simulink model "npc_controller"  (R2022a)
settings: Solver=FixedStepDiscrete  StartTime=0.0  StopTime=20  RelTol=1e-3  EnableMultiTasking=on
values from neighbouring files (symbols this model uses):
  Tsw = 1.5E-5    [param.sldd]
undefined symbols (not defined in the file or in its folder): CAN_O_INT, CANA_BASE, Down, GPTRIP1SEL, GPTRIP2SEL, GPTRIP3SEL, TZ1, TZ2, TZ3, Up
libraries: simulink x153, hdlsllib x90, c2802xlib x34, c2837xDlib x18, c280xlib x12, canmsglib x9, c2838xlib x8, idelinklib_common x3, c2806xlib x2, slpidlib x2, c28004xlib x2, c281xlib x2
(part 39 of 45)

== system npc_controller/IDLE_AND_TIMER/codegen/IDLE/idle_task/report_adc/Subsystem8 ==
  adc : Inport
  zero_offset : Inport  Port=2
  gain : Inport  Port=3
  Product6 : Product  OutDataTypeStr=single
  Saturation : Saturate  UpperLimit=inf  LowerLimit=0
  Subtract : Sum  Inputs=+-  AccumDataTypeStr=single  OutDataTypeStr=single
  actual : Outport
  wires:
  Saturation/1 -> Product6/1
  Subtract/1 -> Saturation/1
  zero_offset/1 -> Subtract/2
  adc/1 -> Subtract/1
  gain/1 -> Product6/2
  Product6/1 -> actual/1

== system npc_controller/IDLE_AND_TIMER/codegen/IDLE/idle_task/report_adc/Subsystem9 ==
  adc : Inport
  gain : Inport  Port=2
  Product6 : Product  OutDataTypeStr=single
  actual : Outport
  wires:
  adc/1 -> Product6/1
  gain/1 -> Product6/2
  Product6/1 -> actual/1

== system npc_controller/IDLE_AND_TIMER/codegen/IDLE/idle_task/report_adc1/Subsystem1 ==
  adc : Inport
  zero_offset : Inport  Port=2
  gain : Inport  Port=3
  Product6 : Product  OutDataTypeStr=single
  Saturation : Saturate  UpperLimit=inf  LowerLimit=0
  Subtract : Sum  Inputs=+-  AccumDataTypeStr=single  OutDataTypeStr=single
  actual : Outport
  wires:
  Product6/1 -> actual/1
  gain/1 -> Product6/2
  adc/1 -> Subtract/1
  zero_offset/1 -> Subtract/2
  Subtract/1 -> Saturation/1
  Saturation/1 -> Product6/1

== system npc_controller/IDLE_AND_TIMER/codegen/IDLE/idle_task/report_adc1/Subsystem10 ==
  adc : Inport
  gain : Inport  Port=2
  Product6 : Product  OutDataTypeStr=single
  actual : Outport
  wires:
  adc/1 -> Product6/1
  gain/1 -> Product6/2
  Product6/1 -> actual/1

== system npc_controller/IDLE_AND_TIMER/codegen/IDLE/idle_task/report_adc1/Subsystem11 ==
  adc : Inport
  zero_offset : Inport  Port=2
  gain : Inport  Port=3
  Product6 : Product  OutDataTypeStr=single
  Saturation : Saturate  UpperLimit=inf  LowerLimit=0
  Subtract : Sum  Inputs=+-  AccumDataTypeStr=single  OutDataTypeStr=single
  actual : Outport
  wires:
  Saturation/1 -> Product6/1
  Subtract/1 -> Saturation/1
  zero_offset/1 -> Subtract/2
  adc/1 -> Subtract/1
  gain/1 -> Product6/2
  Product6/1 -> actual/1

== system npc_controller/IDLE_AND_TIMER/codegen/IDLE/idle_task/report_adc1/Subsystem2 ==
  adc : Inport
  zero_offset : Inport  Port=2
  gain : Inport  Port=3
  Product6 : Product  OutDataTypeStr=single
  Saturation : Saturate  UpperLimit=inf  LowerLimit=0
  Subtract : Sum  Inputs=+-  AccumDataTypeStr=single  OutDataTypeStr=single
  actual : Outport
  wires:
  Saturation/1 -> Product6/1
  Subtract/1 -> Saturation/1
  zero_offset/1 -> Subtract/2
  adc/1 -> Subtract/1
  gain/1 -> Product6/2
  Product6/1 -> actual/1

== system npc_controller/IDLE_AND_TIMER/codegen/IDLE/idle_task/report_adc1/Subsystem3 ==
  adc : Inport
  zero_offset : Inport  Port=2
  gain : Inport  Port=3
  Product6 : Product  OutDataTypeStr=single
  Saturation : Saturate  UpperLimit=inf  LowerLimit=0
  Subtract : Sum  Inputs=+-  AccumDataTypeStr=single  OutDataTypeStr=single
  actual : Outport
  wires:
  Product6/1 -> actual/1
  gain/1 -> Product6/2
  adc/1 -> Subtract/1
  zero_offset/1 -> Subtract/2
  Subtract/1 -> Saturation/1
  Saturation/1 -> Product6/1

== system npc_controller/IDLE_AND_TIMER/codegen/IDLE/idle_task/report_adc1/Subsystem4 ==
  adc : Inport
  zero_offset : Inport  Port=2
  gain : Inport  Port=3
  Product6 : Product  OutDataTypeStr=single
  Saturation : Saturate  UpperLimit=inf  LowerLimit=0
  Subtract : Sum  Inputs=+-  AccumDataTypeStr=single  OutDataTypeStr=single
  actual : Outport
  wires:
  Saturation/1 -> Product6/1
  Subtract/1 -> Saturation/1
  zero_offset/1 -> Subtract/2
  adc/1 -> Subtract/1
  gain/1 -> Product6/2
  Product6/1 -> actual/1

== system npc_controller/IDLE_AND_TIMER/codegen/IDLE/idle_task/report_adc1/Subsystem5 ==
  adc : Inport
  zero_offset : Inport  Port=2
  gain : Inport  Port=3
  Product6 : Product  OutDataTypeStr=single
  Saturation : Saturate  UpperLimit=inf  LowerLimit=0
  Subtract : Sum  Inputs=+-  AccumDataTypeStr=single  OutDataTypeStr=single
  actual : Outport
  wires:
  Product6/1 -> actual/1
  gain/1 -> Product6/2
  adc/1 -> Subtract/1
  zero_offset/1 -> Subtract/2
  Subtract/1 -> Saturation/1
  Saturation/1 -> Product6/1

== system npc_controller/IDLE_AND_TIMER/codegen/IDLE/idle_task/report_adc1/Subsystem6 ==
  adc : Inport
  zero_offset : Inport  Port=2
  gain : Inport  Port=3
  Product6 : Product  OutDataTypeStr=single
  Saturation : Saturate  UpperLimit=inf  LowerLimit=0
  Subtract : Sum  Inputs=+-  AccumDataTypeStr=single  OutDataTypeStr=single
  actual : Outport
  wires:
  Saturation/1 -> Product6/1
  Subtract/1 -> Saturation/1
  zero_offset/1 -> Subtract/2
  adc/1 -> Subtract/1
  gain/1 -> Product6/2
  Product6/1 -> actual/1

== system npc_controller/IDLE_AND_TIMER/codegen/IDLE/idle_task/report_adc1/Subsystem7 ==
  adc : Inport
  zero_offset : Inport  Port=2
  gain : Inport  Port=3
  Product6 : Product  OutDataTypeStr=single
  Saturation : Saturate  UpperLimit=inf  LowerLimit=0
  Subtract : Sum  Inputs=+-  AccumDataTypeStr=single  OutDataTypeStr=single
  actual : Outport
  wires:
  Saturation/1 -> Product6/1
  Subtract/1 -> Saturation/1
  zero_offset/1 -> Subtract/2
  adc/1 -> Subtract/1
  gain/1 -> Product6/2
  Product6/1 -> actual/1

== system npc_controller/IDLE_AND_TIMER/codegen/IDLE/idle_task/report_adc1/Subsystem8 ==
  adc : Inport
  zero_offset : Inport  Port=2
  gain : Inport  Port=3
  Product6 : Product  OutDataTypeStr=single
  Saturation : Saturate  UpperLimit=inf  LowerLimit=0
  Subtract : Sum  Inputs=+-  AccumDataTypeStr=single  OutDataTypeStr=single
  actual : Outport
  wires:
  Product6/1 -> actual/1
  gain/1 -> Product6/2
  adc/1 -> Subtract/1
  zero_offset/1 -> Subtract/2
  Subtract/1 -> Saturation/1
  Saturation/1 -> Product6/1

== system npc_controller/IDLE_AND_TIMER/codegen/IDLE/idle_task/report_adc1/Subsystem9 ==
  adc : Inport
  gain : Inport  Port=2
  Product6 : Product  OutDataTypeStr=single
  actual : Outport
  wires:
  Product6/1 -> actual/1
  gain/1 -> Product6/2
  adc/1 -> Product6/1

== system npc_controller/IDLE_AND_TIMER/codegen/IDLE/idle_task/set_tmp_mux/incr_cnt_tmp_mux ==
  function : TriggerPort  TriggerType=function-call  VariantControl=Variant
  Data Store Read : DataStoreRead  DataStoreName=cnt_tmp_mux  IndexOptions=Index vector (dialog)  Indices=1  OutputSizes=1
  If : If  IfExpression=u1 < 4
  cnt_idle : Subsystem  TreatAsAtomicUnit=on
  cnt_idle_sat : Subsystem  TreatAsAtomicUnit=on
  wires:
  Data Store Read/1 -> If/1
  If/1 -> cnt_idle/Action
  If/2 -> cnt_idle_sat/Action

== system npc_controller/IDLE_AND_TIMER/codegen/IDLE/idle_task/set_tmp_mux/parse_cnt_tmp_mux ==
  function : TriggerPort  TriggerType=function-call  VariantControl=Variant
  Data Store Read : DataStoreRead  DataStoreName=cnt_tmp_mux  IndexOptions=Index vector (dialog)  Indices=1  OutputSizes=1
  Switch Case : SwitchCase  CaseConditions={0, 1, 2, 3}
  cnt_tmp_mux_0 : Subsystem  TreatAsAtomicUnit=on
  cnt_tmp_mux_1 : Subsystem  TreatAsAtomicUnit=on
  cnt_tmp_mux_2 : Subsystem  TreatAsAtomicUnit=on
  cnt_tmp_mux_3 : Subsystem  TreatAsAtomicUnit=on
  wires:
  Data Store Read/1 -> Switch Case/1
  Switch Case/1 -> cnt_tmp_mux_0/Action
  Switch Case/2 -> cnt_tmp_mux_1/Action
  Switch Case/3 -> cnt_tmp_mux_2/Action
  Switch Case/4 -> cnt_tmp_mux_3/Action

== system npc_controller/IDLE_AND_TIMER/codegen/IDLE/idle_task/set_tmp_mux/set_tmp_mux ==
  Trigger : TriggerPort  TriggerType=function-call  VariantControl=(inherit)  PortDimensions=1
  Data Store Read : DataStoreRead  DataStoreName=tmp_mux_s0  IndexOptions=Index vector (dialog)  Indices=1  OutputSizes=1
  Data Store Read1 : DataStoreRead  DataStoreName=tmp_mux_s1  IndexOptions=Index vector (dialog)  Indices=1  OutputSizes=1
  Data Store Read2 : DataStoreRead  DataStoreName=tmp_mux_s2  IndexOptions=Index vector (dialog)  Indices=1  OutputSizes=1
  GPIO63 : c2837xDlib/Digital Output  GPIO_Number=GPIO56~GPIO63  GPIO_Bit0=off  GPIO_BIT0_Toggle=off  GPIO_Bit1=off  GPIO_BIT1_Toggle=off  GPIO_Bit2=off  GPIO_BIT2_Toggle=off  GPIO_Bit3=off  GPIO_BIT3_Toggle=off  GPIO_Bit4=off  GPIO_BIT4_Toggle=off  GPIO_Bit5=off  GPIO_BIT5_Toggle=off  GPIO_Bit6=off  GPIO_BIT6_Toggle=off  GPIO_Bit7=on  GPIO_BIT7_Toggle=off
      settings: SourceProductBaseCode=TIC2000
  GPIO64 : c2837xDlib/Digital Output  GPIO_Number=GPIO64~GPIO71  GPIO_Bit0=on  GPIO_BIT0_Toggle=off  GPIO_Bit1=off  GPIO_BIT1_Toggle=off  GPIO_Bit2=off  GPIO_BIT2_Toggle=off  GPIO_Bit3=off  GPIO_BIT3_Toggle=off  GPIO_Bit4=off  GPIO_BIT4_Toggle=off  GPIO_Bit5=off  GPIO_BIT5_Toggle=off  GPIO_Bit6=off  GPIO_BIT6_Toggle=off  GPIO_Bit7=off  GPIO_BIT7_Toggle=off
      settings: SourceProductBaseCode=TIC2000
  GPIO65 : c2837xDlib/Digital Output  GPIO_Number=GPIO64~GPIO71  GPIO_Bit0=off  GPIO_BIT0_Toggle=off  GPIO_Bit1=on  GPIO_BIT1_Toggle=off  GPIO_Bit2=off  GPIO_BIT2_Toggle=off  GPIO_Bit3=off  GPIO_BIT3_Toggle=off  GPIO_Bit4=off  GPIO_BIT4_Toggle=off  GPIO_Bit5=off  GPIO_BIT5_Toggle=off  GPIO_Bit6=off  GPIO_BIT6_Toggle=off  GPIO_Bit7=off  GPIO_BIT7_Toggle=off
      settings: SourceProductBaseCode=TIC2000
  wires:
  Data Store Read1/1 -> GPIO64/1
  Data Store Read/1 -> GPIO63/1
  Data Store Read2/1 -> GPIO65/1

== system npc_controller/IDLE_AND_TIMER/codegen/IDLE/idle_task1/get_adc_tmp_mux/get_tmp_mux_inlet ==
  In1 : Inport
  Action Port : ActionPort  ActionPortLabel=case [ 3 ]:
  Data Store Write13 : DataStoreWrite  DataStoreName=adc_temp_inlet  IndexOptions=Index vector (dialog)  Indices=1  OutputSizes=1
  wires:
  In1/1 -> Data Store Write13/1

== system npc_controller/IDLE_AND_TIMER/codegen/IDLE/idle_task1/get_adc_tmp_mux/get_tmp_mux_npca ==
  In1 : Inport
  Action Port : ActionPort  ActionPortLabel=case [ 0 ]:
  Data Store Write13 : DataStoreWrite  DataStoreName=adc_temp_npca  IndexOptions=Index vector (dialog)  Indices=1  OutputSizes=1
  wires:
  In1/1 -> Data Store Write13/1

== system npc_controller/IDLE_AND_TIMER/codegen/IDLE/idle_task1/get_adc_tmp_mux/get_tmp_mux_npcb ==
  In1 : Inport
  Action Port : ActionPort  ActionPortLabel=case [ 1 ]:
  Data Store Write13 : DataStoreWrite  DataStoreName=adc_temp_npcb  IndexOptions=Index vector (dialog)  Indices=1  OutputSizes=1
  wires:
  In1/1 -> Data Store Write13/1

== system npc_controller/IDLE_AND_TIMER/codegen/IDLE/idle_task1/get_adc_tmp_mux/get_tmp_mux_npcc ==
  In1 : Inport
  Action Port : ActionPort  ActionPortLabel=case [ 2 ]:
  Data Store Write13 : DataStoreWrite  DataStoreName=adc_temp_npcc  IndexOptions=Index vector (dialog)  Indices=1  OutputSizes=1
  wires:
  In1/1 -> Data Store Write13/1

== system npc_controller/IDLE_AND_TIMER/codegen/IDLE/idle_task1/hkeep/tfv ==
  function : TriggerPort  TriggerType=function-call  VariantControl=Variant
  hkeep1 : Stateflow chart  TreatAsAtomicUnit=on

== system npc_controller/IDLE_AND_TIMER/codegen/IDLE/idle_task1/hkeep/tz ==
  note: reading the tz flag through epwm2 registers and writing to tz_ocp and tz_ovp variables. tz_ocp & tz_ovp are used in state machine
  note: npc_controller_DWork .tz_ocp = EPwm2Regs.TZOSTFLG.bit.OST1;
      | npc_controller_DWork .tz_ovp = EPwm2Regs.TZOSTFLG.bit.OST2;
  function : TriggerPort  TriggerType=function-call  VariantControl=Variant
  System Outputs2 : Subsystem  mask(System Outputs){ShowInLibBrowser=0}
      mask prompts: ShowInLibBrowser "Simulink:masks:CustCodeMaskParam1_MP"
      settings: CopyFcn=cccopyfcn(gcb)  OpenFcn=ccopenfcn('System Outputs Function')
      mask Help: eval('feval(''rtwprivate'',''rtwhelpview'',''rtw_sys_outputs_block'')');
      mask Display: disp('System\nOutputs');

== system npc_controller/IDLE_AND_TIMER/codegen/IDLE/idle_task1/report_adc/Subsystem1 ==
  adc : Inport
  zero_offset : Inport  Port=2
  gain : Inport  Port=3
  Product6 : Product  OutDataTypeStr=single
  Saturation : Saturate  UpperLimit=inf  LowerLimit=0
  Subtract : Sum  Inputs=+-  AccumDataTypeStr=single  OutDataTypeStr=single
  actual : Outport
  wires:
  Saturation/1 -> Product6/1
  Subtract/1 -> Saturation/1
  zero_offset/1 -> Subtract/2
  adc/1 -> Subtract/1
  gain/1 -> Product6/2
  Product6/1 -> actual/1

== system npc_controller/IDLE_AND_TIMER/codegen/IDLE/idle_task1/report_adc/Subsystem10 ==
  adc : Inport
  gain : Inport  Port=2
  Product6 : Product  OutDataTypeStr=single
  actual : Outport
  wires:
  Product6/1 -> actual/1
  gain/1 -> Product6/2
  adc/1 -> Product6/1

== system npc_controller/IDLE_AND_TIMER/codegen/IDLE/idle_task1/report_adc/Subsystem11 ==
  adc : Inport
  zero_offset : Inport  Port=2
  gain : Inport  Port=3
  Product6 : Product  OutDataTypeStr=single
  Saturation : Saturate  UpperLimit=inf  LowerLimit=0
  Subtract : Sum  Inputs=+-  AccumDataTypeStr=single  OutDataTypeStr=single
  actual : Outport
  wires:
  Product6/1 -> actual/1
  gain/1 -> Product6/2
  adc/1 -> Subtract/1
  zero_offset/1 -> Subtract/2
  Subtract/1 -> Saturation/1
  Saturation/1 -> Product6/1

== system npc_controller/IDLE_AND_TIMER/codegen/IDLE/idle_task1/report_adc/Subsystem2 ==
  adc : Inport
  zero_offset : Inport  Port=2
  gain : Inport  Port=3
  Product6 : Product  OutDataTypeStr=single
  Saturation : Saturate  UpperLimit=inf  LowerLimit=0
  Subtract : Sum  Inputs=+-  AccumDataTypeStr=single  OutDataTypeStr=single
  actual : Outport
  wires:
  Product6/1 -> actual/1
  gain/1 -> Product6/2
  adc/1 -> Subtract/1
  zero_offset/1 -> Subtract/2
  Subtract/1 -> Saturation/1
  Saturation/1 -> Product6/1

== system npc_controller/IDLE_AND_TIMER/codegen/IDLE/idle_task1/report_adc/Subsystem3 ==
  adc : Inport
  zero_offset : Inport  Port=2
  gain : Inport  Port=3
  Product6 : Product  OutDataTypeStr=single
  Saturation : Saturate  UpperLimit=inf  LowerLimit=0
  Subtract : Sum  Inputs=+-  AccumDataTypeStr=single  OutDataTypeStr=single
  actual : Outport
  wires:
  Saturation/1 -> Product6/1
  Subtract/1 -> Saturation/1
  zero_offset/1 -> Subtract/2
  adc/1 -> Subtract/1
  gain/1 -> Product6/2
  Product6/1 -> actual/1

== system npc_controller/IDLE_AND_TIMER/codegen/IDLE/idle_task1/report_adc/Subsystem4 ==
  adc : Inport
  zero_offset : Inport  Port=2
  gain : Inport  Port=3
  Product6 : Product  OutDataTypeStr=single
  Saturation : Saturate  UpperLimit=inf  LowerLimit=0
  Subtract : Sum  Inputs=+-  AccumDataTypeStr=single  OutDataTypeStr=single
  actual : Outport
  wires:
  Product6/1 -> actual/1
  gain/1 -> Product6/2
  adc/1 -> Subtract/1
  zero_offset/1 -> Subtract/2
  Subtract/1 -> Saturation/1
  Saturation/1 -> Product6/1

== system npc_controller/IDLE_AND_TIMER/codegen/IDLE/idle_task1/report_adc/Subsystem5 ==
  adc : Inport
  zero_offset : Inport  Port=2
  gain : Inport  Port=3
  Product6 : Product  OutDataTypeStr=single
  Saturation : Saturate  UpperLimit=inf  LowerLimit=0
  Subtract : Sum  Inputs=+-  AccumDataTypeStr=single  OutDataTypeStr=single
  actual : Outport
  wires:
  Saturation/1 -> Product6/1
  Subtract/1 -> Saturation/1
  zero_offset/1 -> Subtract/2
  adc/1 -> Subtract/1
  gain/1 -> Product6/2
  Product6/1 -> actual/1

== system npc_controller/IDLE_AND_TIMER/codegen/IDLE/idle_task1/report_adc/Subsystem6 ==
  adc : Inport
  zero_offset : Inport  Port=2
  gain : Inport  Port=3
  Product6 : Product  OutDataTypeStr=single
  Saturation : Saturate  UpperLimit=inf  LowerLimit=0
  Subtract : Sum  Inputs=+-  AccumDataTypeStr=single  OutDataTypeStr=single
  actual : Outport
  wires:
  Product6/1 -> actual/1
  gain/1 -> Product6/2
  adc/1 -> Subtract/1
  zero_offset/1 -> Subtract/2
  Subtract/1 -> Saturation/1
  Saturation/1 -> Product6/1

== system npc_controller/IDLE_AND_TIMER/codegen/IDLE/idle_task1/report_adc/Subsystem7 ==
  adc : Inport
  zero_offset : Inport  Port=2
  gain : Inport  Port=3
  Product6 : Product  OutDataTypeStr=single
  Saturation : Saturate  UpperLimit=inf  LowerLimit=0
  Subtract : Sum  Inputs=+-  AccumDataTypeStr=single  OutDataTypeStr=single
  actual : Outport
  wires:
  Product6/1 -> actual/1
  gain/1 -> Product6/2
  adc/1 -> Subtract/1
  zero_offset/1 -> Subtract/2
  Subtract/1 -> Saturation/1
  Saturation/1 -> Product6/1

== system npc_controller/IDLE_AND_TIMER/codegen/IDLE/idle_task1/report_adc/Subsystem8 ==
  adc : Inport
  zero_offset : Inport  Port=2
  gain : Inport  Port=3
  Product6 : Product  OutDataTypeStr=single
  Saturation : Saturate  UpperLimit=inf  LowerLimit=0
  Subtract : Sum  Inputs=+-  AccumDataTypeStr=single  OutDataTypeStr=single
  actual : Outport
  wires:
  Saturation/1 -> Product6/1
  Subtract/1 -> Saturation/1
  zero_offset/1 -> Subtract/2
  adc/1 -> Subtract/1
  gain/1 -> Product6/2
  Product6/1 -> actual/1

== system npc_controller/IDLE_AND_TIMER/codegen/IDLE/idle_task1/report_adc/Subsystem9 ==
  adc : Inport
  gain : Inport  Port=2
  Product6 : Product  OutDataTypeStr=single
  actual : Outport
  wires:
  adc/1 -> Product6/1
  gain/1 -> Product6/2
  Product6/1 -> actual/1

== system npc_controller/IDLE_AND_TIMER/codegen/IDLE/idle_task1/report_adc1/Subsystem1 ==
  adc : Inport
  zero_offset : Inport  Port=2
  gain : Inport  Port=3
  Product6 : Product  OutDataTypeStr=single
  Saturation : Saturate  UpperLimit=inf  LowerLimit=0
  Subtract : Sum  Inputs=+-  AccumDataTypeStr=single  OutDataTypeStr=single
  actual : Outport
  wires:
  Product6/1 -> actual/1
  gain/1 -> Product6/2
  adc/1 -> Subtract/1
  zero_offset/1 -> Subtract/2
  Subtract/1 -> Saturation/1
  Saturation/1 -> Product6/1

== system npc_controller/IDLE_AND_TIMER/codegen/IDLE/idle_task1/report_adc1/Subsystem10 ==
  adc : Inport
  gain : Inport  Port=2
  Product6 : Product  OutDataTypeStr=single
  actual : Outport
  wires:
  adc/1 -> Product6/1
  gain/1 -> Product6/2
  Product6/1 -> actual/1

== system npc_controller/IDLE_AND_TIMER/codegen/IDLE/idle_task1/report_adc1/Subsystem11 ==
  adc : Inport
  zero_offset : Inport  Port=2
  gain : Inport  Port=3
  Product6 : Product  OutDataTypeStr=single
  Saturation : Saturate  UpperLimit=inf  LowerLimit=0
  Subtract : Sum  Inputs=+-  AccumDataTypeStr=single  OutDataTypeStr=single
  actual : Outport
  wires:
  Saturation/1 -> Product6/1
  Subtract/1 -> Saturation/1
  zero_offset/1 -> Subtract/2
  adc/1 -> Subtract/1
  gain/1 -> Product6/2
  Product6/1 -> actual/1

== system npc_controller/IDLE_AND_TIMER/codegen/IDLE/idle_task1/report_adc1/Subsystem2 ==
  adc : Inport
  zero_offset : Inport  Port=2
  gain : Inport  Port=3
  Product6 : Product  OutDataTypeStr=single
  Saturation : Saturate  UpperLimit=inf  LowerLimit=0
  Subtract : Sum  Inputs=+-  AccumDataTypeStr=single  OutDataTypeStr=single
  actual : Outport
  wires:
  Saturation/1 -> Product6/1
  Subtract/1 -> Saturation/1
  zero_offset/1 -> Subtract/2
  adc/1 -> Subtract/1
  gain/1 -> Product6/2
  Product6/1 -> actual/1

== system npc_controller/IDLE_AND_TIMER/codegen/IDLE/idle_task1/report_adc1/Subsystem3 ==
  adc : Inport
  zero_offset : Inport  Port=2
  gain : Inport  Port=3
  Product6 : Product  OutDataTypeStr=single
  Saturation : Saturate  UpperLimit=inf  LowerLimit=0
  Subtract : Sum  Inputs=+-  AccumDataTypeStr=single  OutDataTypeStr=single
  actual : Outport
  wires:
  Product6/1 -> actual/1
  gain/1 -> Product6/2
  adc/1 -> Subtract/1
  zero_offset/1 -> Subtract/2
  Subtract/1 -> Saturation/1
  Saturation/1 -> Product6/1

== system npc_controller/IDLE_AND_TIMER/codegen/IDLE/idle_task1/report_adc1/Subsystem4 ==
  adc : Inport
  zero_offset : Inport  Port=2
  gain : Inport  Port=3
  Product6 : Product  OutDataTypeStr=single
  Saturation : Saturate  UpperLimit=inf  LowerLimit=0
  Subtract : Sum  Inputs=+-  AccumDataTypeStr=single  OutDataTypeStr=single
  actual : Outport
  wires:
  Saturation/1 -> Product6/1
  Subtract/1 -> Saturation/1
  zero_offset/1 -> Subtract/2
  adc/1 -> Subtract/1
  gain/1 -> Product6/2
  Product6/1 -> actual/1

== system npc_controller/IDLE_AND_TIMER/codegen/IDLE/idle_task1/report_adc1/Subsystem5 ==
  adc : Inport
  zero_offset : Inport  Port=2
  gain : Inport  Port=3
  Product6 : Product  OutDataTypeStr=single
  Saturation : Saturate  UpperLimit=inf  LowerLimit=0
  Subtract : Sum  Inputs=+-  AccumDataTypeStr=single  OutDataTypeStr=single
  actual : Outport
  wires:
  Product6/1 -> actual/1
  gain/1 -> Product6/2
  adc/1 -> Subtract/1
  zero_offset/1 -> Subtract/2
  Subtract/1 -> Saturation/1
  Saturation/1 -> Product6/1

== system npc_controller/IDLE_AND_TIMER/codegen/IDLE/idle_task1/report_adc1/Subsystem6 ==
  adc : Inport
  zero_offset : Inport  Port=2
  gain : Inport  Port=3
  Product6 : Product  OutDataTypeStr=single
  Saturation : Saturate  UpperLimit=inf  LowerLimit=0
  Subtract : Sum  Inputs=+-  AccumDataTypeStr=single  OutDataTypeStr=single
  actual : Outport
  wires:
  Saturation/1 -> Product6/1
  Subtract/1 -> Saturation/1
  zero_offset/1 -> Subtract/2
  adc/1 -> Subtract/1
  gain/1 -> Product6/2
  Product6/1 -> actual/1

== system npc_controller/IDLE_AND_TIMER/codegen/IDLE/idle_task1/report_adc1/Subsystem7 ==
  adc : Inport
  zero_offset : Inport  Port=2
  gain : Inport  Port=3
  Product6 : Product  OutDataTypeStr=single
  Saturation : Saturate  UpperLimit=inf  LowerLimit=0
  Subtract : Sum  Inputs=+-  AccumDataTypeStr=single  OutDataTypeStr=single
  actual : Outport
  wires:
  Saturation/1 -> Product6/1
  Subtract/1 -> Saturation/1
  zero_offset/1 -> Subtract/2
  adc/1 -> Subtract/1
  gain/1 -> Product6/2
  Product6/1 -> actual/1

== system npc_controller/IDLE_AND_TIMER/codegen/IDLE/idle_task1/report_adc1/Subsystem8 ==
  adc : Inport
  zero_offset : Inport  Port=2
  gain : Inport  Port=3
  Product6 : Product  OutDataTypeStr=single
  Saturation : Saturate  UpperLimit=inf  LowerLimit=0
  Subtract : Sum  Inputs=+-  AccumDataTypeStr=single  OutDataTypeStr=single
  actual : Outport
  wires:
  Product6/1 -> actual/1
  gain/1 -> Product6/2
  adc/1 -> Subtract/1
  zero_offset/1 -> Subtract/2
  Subtract/1 -> Saturation/1
  Saturation/1 -> Product6/1

== system npc_controller/IDLE_AND_TIMER/codegen/IDLE/idle_task1/report_adc1/Subsystem9 ==
  adc : Inport
  gain : Inport  Port=2
  Product6 : Product  OutDataTypeStr=single
  actual : Outport
  wires:
  Product6/1 -> actual/1
  gain/1 -> Product6/2
  adc/1 -> Product6/1

== system npc_controller/IDLE_AND_TIMER/codegen/IDLE/idle_task1/set_tmp_mux/incr_cnt_tmp_mux ==
  function : TriggerPort  TriggerType=function-call  VariantControl=Variant
  Data Store Read : DataStoreRead  DataStoreName=cnt_tmp_mux  IndexOptions=Index vector (dialog)  Indices=1  OutputSizes=1
  If : If  IfExpression=u1 < 4
  cnt_idle : Subsystem  TreatAsAtomicUnit=on
  cnt_idle_sat : Subsystem  TreatAsAtomicUnit=on
  wires:
  Data Store Read/1 -> If/1
  If/1 -> cnt_idle/Action
  If/2 -> cnt_idle_sat/Action

== system npc_controller/IDLE_AND_TIMER/codegen/IDLE/idle_task1/set_tmp_mux/parse_cnt_tmp_mux ==
  function : TriggerPort  TriggerType=function-call  VariantControl=Variant
  Data Store Read : DataStoreRead  DataStoreName=cnt_tmp_mux  IndexOptions=Index vector (dialog)  Indices=1  OutputSizes=1
  Switch Case : SwitchCase  CaseConditions={0, 1, 2, 3}
  cnt_tmp_mux_0 : Subsystem  TreatAsAtomicUnit=on
  cnt_tmp_mux_1 : Subsystem  TreatAsAtomicUnit=on
  cnt_tmp_mux_2 : Subsystem  TreatAsAtomicUnit=on
  cnt_tmp_mux_3 : Subsystem  TreatAsAtomicUnit=on
  wires:
  Data Store Read/1 -> Switch Case/1
  Switch Case/1 -> cnt_tmp_mux_0/Action
  Switch Case/2 -> cnt_tmp_mux_1/Action
  Switch Case/3 -> cnt_tmp_mux_2/Action
  Switch Case/4 -> cnt_tmp_mux_3/Action

== system npc_controller/IDLE_AND_TIMER/codegen/IDLE/idle_task1/set_tmp_mux/set_tmp_mux ==
  Trigger : TriggerPort  TriggerType=function-call  VariantControl=(inherit)  PortDimensions=1
  Data Store Read : DataStoreRead  DataStoreName=tmp_mux_s0  IndexOptions=Index vector (dialog)  Indices=1  OutputSizes=1
  Data Store Read1 : DataStoreRead  DataStoreName=tmp_mux_s1  IndexOptions=Index vector (dialog)  Indices=1  OutputSizes=1
  Data Store Read2 : DataStoreRead  DataStoreName=tmp_mux_s2  IndexOptions=Index vector (dialog)  Indices=1  OutputSizes=1
  GPIO63 : c2837xDlib/Digital Output  GPIO_Number=GPIO56~GPIO63  GPIO_Bit0=off  GPIO_BIT0_Toggle=off  GPIO_Bit1=off  GPIO_BIT1_Toggle=off  GPIO_Bit2=off  GPIO_BIT2_Toggle=off  GPIO_Bit3=off  GPIO_BIT3_Toggle=off  GPIO_Bit4=off  GPIO_BIT4_Toggle=off  GPIO_Bit5=off  GPIO_BIT5_Toggle=off  GPIO_Bit6=off  GPIO_BIT6_Toggle=off  GPIO_Bit7=on  GPIO_BIT7_Toggle=off
      settings: SourceProductBaseCode=TIC2000
  GPIO64 : c2837xDlib/Digital Output  GPIO_Number=GPIO64~GPIO71  GPIO_Bit0=on  GPIO_BIT0_Toggle=off  GPIO_Bit1=off  GPIO_BIT1_Toggle=off  GPIO_Bit2=off  GPIO_BIT2_Toggle=off  GPIO_Bit3=off  GPIO_BIT3_Toggle=off  GPIO_Bit4=off  GPIO_BIT4_Toggle=off  GPIO_Bit5=off  GPIO_BIT5_Toggle=off  GPIO_Bit6=off  GPIO_BIT6_Toggle=off  GPIO_Bit7=off  GPIO_BIT7_Toggle=off
      settings: SourceProductBaseCode=TIC2000
  GPIO65 : c2837xDlib/Digital Output  GPIO_Number=GPIO64~GPIO71  GPIO_Bit0=off  GPIO_BIT0_Toggle=off  GPIO_Bit1=on  GPIO_BIT1_Toggle=off  GPIO_Bit2=off  GPIO_BIT2_Toggle=off  GPIO_Bit3=off  GPIO_BIT3_Toggle=off  GPIO_Bit4=off  GPIO_BIT4_Toggle=off  GPIO_Bit5=off  GPIO_BIT5_Toggle=off  GPIO_Bit6=off  GPIO_BIT6_Toggle=off  GPIO_Bit7=off  GPIO_BIT7_Toggle=off
      settings: SourceProductBaseCode=TIC2000
  wires:
  Data Store Read1/1 -> GPIO64/1
  Data Store Read/1 -> GPIO63/1
  Data Store Read2/1 -> GPIO65/1

== system npc_controller/CONTROL/CONTROL/false/CLA_CONTROL/CONTROL/pwm_generation1/Subsystem ==
  note: Note:
      | pol_pha
      | 0 - pos
      | 1 - neg
  pol : Inport
  pwm_s1 : Inport  Port=2
  pwm_s4 : Inport  Port=3
  Cast To Single : DataTypeConversion  OutDataTypeStr=uint8  SaturateOnIntegerOverflow=off  RndMeth=Floor
  If : If  IfExpression=u1 == 0
  If Action Subsystem : Subsystem  TreatAsAtomicUnit=on
  If Action Subsystem1 : Subsystem  TreatAsAtomicUnit=on
  Merge : Merge
  epwm1b : Outport
  wires:
  pol/1 -> Cast To Single/1
  If/2 -> If Action Subsystem1/Action
  If/1 -> If Action Subsystem/Action
  If Action Subsystem1/1(Out1) -> Merge/2
  If Action Subsystem/1(Out1) -> Merge/1
  Merge/1 -> epwm1b/1
  pwm_s1/1 -> If Action Subsystem/1(In1)
  pwm_s4/1 -> If Action Subsystem1/1(In1)
  Cast To Single/1 -> If/1

== system npc_controller/CONTROL/CONTROL/false/CLA_CONTROL/CONTROL/pwm_generation1/Subsystem1 ==
  note: Note:
      | pol_pha
      | 0 - pos
      | 1 - neg
  pol : Inport
  pwm_s1 : Inport  Port=2
  pwm_s4 : Inport  Port=3
  Cast To Single : DataTypeConversion  OutDataTypeStr=uint8  SaturateOnIntegerOverflow=off  RndMeth=Floor
  If : If  IfExpression=u1 == 0
  If Action Subsystem : Subsystem  TreatAsAtomicUnit=on
  If Action Subsystem1 : Subsystem  TreatAsAtomicUnit=on
  Merge : Merge
  epwm1b : Outport
  wires:
  Cast To Single/1 -> If/1
  pwm_s4/1 -> If Action Subsystem1/1(In1)
  pwm_s1/1 -> If Action Subsystem/1(In1)
  Merge/1 -> epwm1b/1
  If Action Subsystem/1(Out1) -> Merge/1
  If Action Subsystem1/1(Out1) -> Merge/2
  If/1 -> If Action Subsystem/Action
  If/2 -> If Action Subsystem1/Action
  pol/1 -> Cast To Single/1

== system npc_controller/CONTROL/CONTROL/false/CLA_CONTROL/CONTROL/pwm_generation1/Subsystem2 ==
  note: Note:
      | pol_pha
      | 0 - pos
      | 1 - neg
  pol : Inport
  pwm_s1 : Inport  Port=2
  pwm_s4 : Inport  Port=3
  Cast To Single : DataTypeConversion  OutDataTypeStr=uint8  SaturateOnIntegerOverflow=off  RndMeth=Floor
  If : If  IfExpression=u1 == 0
  If Action Subsystem : Subsystem  TreatAsAtomicUnit=on
  If Action Subsystem1 : Subsystem  TreatAsAtomicUnit=on
  Merge : Merge
  epwm1b : Outport
  wires:
  pol/1 -> Cast To Single/1
  If/2 -> If Action Subsystem1/Action
  If/1 -> If Action Subsystem/Action
  If Action Subsystem1/1(Out1) -> Merge/2
  If Action Subsystem/1(Out1) -> Merge/1
  Merge/1 -> epwm1b/1
  pwm_s1/1 -> If Action Subsystem/1(In1)
  pwm_s4/1 -> If Action Subsystem1/1(In1)
  Cast To Single/1 -> If/1

== system npc_controller/CONTROL/CONTROL/false/CLA_CONTROL/CONTROL/pwm_generation1/min_duty ==
  cmp : Inport
  Duty0Pct : Subsystem  TreatAsAtomicUnit=on
  Duty5Pct : Subsystem  TreatAsAtomicUnit=on
  If : If  IfExpression=u1 > 76
  Merge : Merge
  cmp_out : Outport
  wires:
  cmp/1 -> Duty5Pct/1(In1), If/1
  Duty0Pct/1(Out1) -> Merge/2
  If/2 -> Duty0Pct/Action
  Duty5Pct/1(Out1) -> Merge/1
  Merge/1 -> cmp_out/1
  If/1 -> Duty5Pct/Action

== system npc_controller/CONTROL/CONTROL/false/CLA_CONTROL/CONTROL/pwm_generation1/min_duty1 ==
  cmp : Inport
  Duty0Pct : Subsystem  TreatAsAtomicUnit=on
  Duty5Pct : Subsystem  TreatAsAtomicUnit=on
  If : If  IfExpression=u1 > 76
  Merge : Merge
  cmp_out : Outport
  wires:
  If/1 -> Duty5Pct/Action
  Merge/1 -> cmp_out/1
  Duty5Pct/1(Out1) -> Merge/1
  If/2 -> Duty0Pct/Action
  Duty0Pct/1(Out1) -> Merge/2
  cmp/1 -> If/1, Duty5Pct/1(In1)

== system npc_controller/CONTROL/CONTROL/false/CLA_CONTROL/CONTROL/pwm_generation1/min_duty2 ==
  cmp : Inport
  Duty0Pct : Subsystem  TreatAsAtomicUnit=on
  Duty5Pct : Subsystem  TreatAsAtomicUnit=on
  If : If  IfExpression=u1 > 76
  Merge : Merge
  cmp_out : Outport
  wires:
  cmp/1 -> Duty5Pct/1(In1), If/1
  Duty0Pct/1(Out1) -> Merge/2
  If/2 -> Duty0Pct/Action
  Duty5Pct/1(Out1) -> Merge/1
  Merge/1 -> cmp_out/1
  If/1 -> Duty5Pct/Action

== system npc_controller/CONTROL/GET_ADC/ADC/codegen/ADCA/Subsystem6/If Action Subsystem ==
  Action Port : ActionPort  ActionPortLabel=if((u1 > 2979) | (u1 < 1525))
  Constant : Constant  OutDataTypeStr=boolean  SampleTime=-1
  Data Store Write1 : DataStoreWrite  DataStoreName=tfv_iphasec  IndexOptions=Index vector (dialog)  Indices=1  OutputSizes=1
  wires:
  Constant/1 -> Data Store Write1/1

== system npc_controller/CONTROL/GET_ADC/ADC/codegen/ADCA/Subsystem6/If Action Subsystem1 ==
  note: +-30Apeak
  note: //3221 = 40A , 1283 = -40A
  Input : Inport
  Action Port : ActionPort  ActionPortLabel=else
  If Action Subsystem : Subsystem  TreatAsAtomicUnit=on
  If1 : If  Commented=on  IfExpression=(u1 > 2979) | (u1 < 1525)
  If2 : If  IfExpression=(u1 > 3221) | (u1 < 1283)
  wires:
  If2/1 -> If Action Subsystem/Action
  Input/1 -> If2/1

== system npc_controller/CONTROL/GET_ADC/ADC/codegen/ADCA/Subsystem6/If Action Subsystem2 ==
  note: -+60Apeak
  Input : Inport
  Action Port : ActionPort  ActionPortLabel=if(u1 == 0)
  If : If  IfExpression=(u1 > 3705) | (u1 < 798)
  If Action Subsystem : Subsystem  TreatAsAtomicUnit=on
  wires:
  Input/1 -> If/1
  If/1 -> If Action Subsystem/Action

== system npc_controller/CONTROL/GET_ADC/ADC/codegen/ADCA/Subsystem6/calib ==
  note: y = 1.0377x - 68.775
  adc : Inport
  Add : Sum  AccumDataTypeStr=single  OutDataTypeStr=single
  Constant1 : Constant  Value=1.0377  OutDataTypeStr=single
  Constant2 : Constant  Value=-68.775  OutDataTypeStr=single
  Product : Product  OutDataTypeStr=single
  adc_calib : Outport
  wires:
  adc/1 -> Product/1
  Constant1/1 -> Product/2
  Product/1 -> Add/1
  Constant2/1 -> Add/2
  Add/1 -> adc_calib/1

== system npc_controller/CONTROL/GET_ADC/ADC/codegen/ADCA/Subsystem7/If Action Subsystem ==
  Action Port : ActionPort  ActionPortLabel=if((u1 > 2979) | (u1 < 1525))
  Constant : Constant  OutDataTypeStr=boolean  SampleTime=-1
  Data Store Write1 : DataStoreWrite  DataStoreName=tfv_iphaseb  IndexOptions=Index vector (dialog)  Indices=1  OutputSizes=1
  wires:
  Constant/1 -> Data Store Write1/1

== system npc_controller/CONTROL/GET_ADC/ADC/codegen/ADCA/Subsystem7/If Action Subsystem1 ==
  note: +-30Apeak
  note: //3221 = 40A , 1283 = -40A
  Input : Inport
  Action Port : ActionPort  ActionPortLabel=else
  If Action Subsystem : Subsystem  TreatAsAtomicUnit=on
  If1 : If  Commented=on  IfExpression=(u1 > 2979) | (u1 < 1525)
  If2 : If  IfExpression=(u1 > 3221) | (u1 < 1283)
  wires:
  If2/1 -> If Action Subsystem/Action
  Input/1 -> If2/1

== system npc_controller/CONTROL/GET_ADC/ADC/codegen/ADCA/Subsystem7/If Action Subsystem2 ==
  note: -+60Apeak
  Input : Inport
  Action Port : ActionPort  ActionPortLabel=if(u1 == 0)
  If : If  IfExpression=(u1 > 3705) | (u1 < 798)
  If Action Subsystem : Subsystem  TreatAsAtomicUnit=on
  wires:
  Input/1 -> If/1
  If/1 -> If Action Subsystem/Action

== system npc_controller/CONTROL/GET_ADC/ADC/codegen/ADCA/Subsystem7/calib ==
  note: y = 1.0208x - 29.621
  adc : Inport
  Add : Sum  AccumDataTypeStr=single  OutDataTypeStr=single
  Constant1 : Constant  Value=1.02308  OutDataTypeStr=single
  Constant2 : Constant  Value=-29.621  OutDataTypeStr=single
  Product : Product  OutDataTypeStr=single
  adc_calib : Outport
  wires:
  adc/1 -> Product/1
  Constant1/1 -> Product/2
  Product/1 -> Add/1
  Constant2/1 -> Add/2
  Add/1 -> adc_calib/1

== system npc_controller/CONTROL/GET_ADC/ADC/codegen/ADCA/Subsystem8/If Action Subsystem1 ==
  note: +-30Apeak
  note: //3221 = 40A , 1283 = -40A
  Input : Inport
  Action Port : ActionPort  ActionPortLabel=else
  If Action Subsystem : Subsystem  TreatAsAtomicUnit=on
  If1 : If  Commented=on  IfExpression=(u1 > 2979) | (u1 < 1525)
  If2 : If  IfExpression=(u1 > 3221) | (u1 < 1283)
  wires:
  If2/1 -> If Action Subsystem/Action
  Input/1 -> If2/1

== system npc_controller/CONTROL/GET_ADC/ADC/codegen/ADCA/Subsystem8/If Action Subsystem2 ==
  note: -+60Apeak
  Input : Inport
  Action Port : ActionPort  ActionPortLabel=if(u1 == 0)
  If : If  IfExpression=(u1 > 3705) | (u1 < 798)
  If Action Subsystem : Subsystem  TreatAsAtomicUnit=on
  wires:
  Input/1 -> If/1
  If/1 -> If Action Subsystem/Action

== system npc_controller/CONTROL/GET_ADC/ADC/codegen/ADCA/Subsystem8/calib ==
  note: y = 0.9897x + 34.749
  adc : Inport
  Add : Sum  AccumDataTypeStr=single  OutDataTypeStr=single
  Constant1 : Constant  Value=0.9897  OutDataTypeStr=single
  Constant2 : Constant  Value=34.749  OutDataTypeStr=single
  Product : Product  OutDataTypeStr=single
  adc_calib : Outport
  wires:
  adc/1 -> Product/1
  Constant1/1 -> Product/2
  Product/1 -> Add/1
  Constant2/1 -> Add/2
  Add/1 -> adc_calib/1

== system npc_controller/CONTROL/STATE-MACHINE/CPU_CONTROL_100_A2_precharge_pfc_ok2/configGrid/FORCE_TZ/1P/ALL_LEGS/System Outputs2 ==

== system npc_controller/CONTROL/STATE-MACHINE/CPU_CONTROL_100_A2_precharge_pfc_ok2/configGrid/FORCE_TZ/1P/LEG_A/System Outputs2 ==

== system npc_controller/CONTROL/STATE-MACHINE/CPU_CONTROL_100_A2_precharge_pfc_ok2/configGrid/FORCE_TZ/1P/LEG_B/System Outputs2 ==

== system npc_controller/CONTROL/STATE-MACHINE/CPU_CONTROL_100_A2_precharge_pfc_ok2/configGrid/FORCE_TZ/1P/LEG_C/System Outputs2 ==

== system npc_controller/CONTROL/STATE-MACHINE/CPU_CONTROL_100_A2_precharge_pfc_ok2/updatePll3p/PLL/SRF_PLL/Integrator/Accumulation ==
  In1 : Inport  OutDataTypeStr=single
  Action Port : ActionPort
  Out : Outport  OutDataTypeStr=single
  wires:
  In1/1 -> Out/1

== system npc_controller/CONTROL/STATE-MACHINE/CPU_CONTROL_100_A2_precharge_pfc_ok2/updatePll3p/PLL/SRF_PLL/Integrator/Reset Integrator ==
  Action Port : ActionPort
  Constant1 : Constant  Value=0  OutDataTypeStr=single
  Out : Outport
  wires:
  Constant1/1 -> Out/1

== system npc_controller/CONTROL/STATE-MACHINE/CPU_CONTROL_200_A2_precharge_pfc_ok2/configGrid/FORCE_TZ/1P/ALL_LEGS/System Outputs2 ==

== system npc_controller/CONTROL/STATE-MACHINE/CPU_CONTROL_200_A2_precharge_pfc_ok2/configGrid/FORCE_TZ/1P/LEG_A/System Outputs2 ==

== system npc_controller/CONTROL/STATE-MACHINE/CPU_CONTROL_200_A2_precharge_pfc_ok2/configGrid/FORCE_TZ/1P/LEG_B/System Outputs2 ==

== system npc_controller/CONTROL/STATE-MACHINE/CPU_CONTROL_200_A2_precharge_pfc_ok2/configGrid/FORCE_TZ/1P/LEG_C/System Outputs2 ==

== system npc_controller/CONTROL/STATE-MACHINE/CPU_CONTROL_200_A2_precharge_pfc_ok2/updatePll3p/PLL/SRF_PLL/Integrator/Accumulation ==
  In1 : Inport  OutDataTypeStr=single
  Action Port : ActionPort
  Out : Outport  OutDataTypeStr=single
  wires:
  In1/1 -> Out/1

== system npc_controller/CONTROL/STATE-MACHINE/CPU_CONTROL_200_A2_precharge_pfc_ok2/updatePll3p/PLL/SRF_PLL/Integrator/Reset Integrator ==
  Action Port : ActionPort
  Constant1 : Constant  Value=0  OutDataTypeStr=single
  Out : Outport
  wires:
  Constant1/1 -> Out/1

== system npc_controller/CONTROL/STATE-MACHINE/CPU_CONTROL_200_A2_precharge_pfc_ok2_OL SS/configGrid/FORCE_TZ/1P/ALL_LEGS/System Outputs2 ==

== system npc_controller/CONTROL/STATE-MACHINE/CPU_CONTROL_200_A2_precharge_pfc_ok2_OL SS/configGrid/FORCE_TZ/1P/LEG_A/System Outputs2 ==

== system npc_controller/CONTROL/STATE-MACHINE/CPU_CONTROL_200_A2_precharge_pfc_ok2_OL SS/configGrid/FORCE_TZ/1P/LEG_B/System Outputs2 ==

== system npc_controller/CONTROL/STATE-MACHINE/CPU_CONTROL_200_A2_precharge_pfc_ok2_OL SS/configGrid/FORCE_TZ/1P/LEG_C/System Outputs2 ==

== system npc_controller/CONTROL/STATE-MACHINE/CPU_CONTROL_200_A2_precharge_pfc_ok2_OL SS/updatePll3p/PLL/SRF_PLL/Integrator/Accumulation ==
  In1 : Inport  OutDataTypeStr=single
  Action Port : ActionPort
  Out : Outport  OutDataTypeStr=single
  wires:
  In1/1 -> Out/1

== system npc_controller/CONTROL/STATE-MACHINE/CPU_CONTROL_200_A2_precharge_pfc_ok2_OL SS/updatePll3p/PLL/SRF_PLL/Integrator/Reset Integrator ==
  Action Port : ActionPort
  Constant1 : Constant  Value=0  OutDataTypeStr=single
  Out : Outport
  wires:
  Constant1/1 -> Out/1

== system npc_controller/CONTROL/STATE-MACHINE/CPU_CONTROL_200_A2_precharge_pfc_ok2_OL SS2/configGrid/FORCE_TZ/1P/ALL_LEGS/System Outputs2 ==

== system npc_controller/CONTROL/STATE-MACHINE/CPU_CONTROL_200_A2_precharge_pfc_ok2_OL SS2/configGrid/FORCE_TZ/1P/LEG_A/System Outputs2 ==

== system npc_controller/CONTROL/STATE-MACHINE/CPU_CONTROL_200_A2_precharge_pfc_ok2_OL SS2/configGrid/FORCE_TZ/1P/LEG_B/System Outputs2 ==

== system npc_controller/CONTROL/STATE-MACHINE/CPU_CONTROL_200_A2_precharge_pfc_ok2_OL SS2/configGrid/FORCE_TZ/1P/LEG_C/System Outputs2 ==

== system npc_controller/CONTROL/STATE-MACHINE/CPU_CONTROL_200_A2_precharge_pfc_ok2_OL SS2/updatePll3p/PLL/SRF_PLL/Integrator/Accumulation ==
  In1 : Inport  OutDataTypeStr=single
  Action Port : ActionPort
  Out : Outport  OutDataTypeStr=single
  wires:
  In1/1 -> Out/1

== system npc_controller/CONTROL/STATE-MACHINE/CPU_CONTROL_200_A2_precharge_pfc_ok2_OL SS2/updatePll3p/PLL/SRF_PLL/Integrator/Reset Integrator ==
  Action Port : ActionPort
  Constant1 : Constant  Value=0  OutDataTypeStr=single
  Out : Outport
  wires:
  Constant1/1 -> Out/1

== system npc_controller/CONTROL/STATE-MACHINE/CPU_CONTROL_200_A2_precharge_pfc_ok2_OL SS2/updateSequencePhA/pol_vxn1/neg/SR OFF/System Outputs1 ==

== system npc_controller/CONTROL/STATE-MACHINE/CPU_CONTROL_200_A2_precharge_pfc_ok2_OL SS2/updateSequencePhA/pol_vxn1/neg/SR OFF/System Outputs2 ==

== system npc_controller/CONTROL/STATE-MACHINE/CPU_CONTROL_200_A2_precharge_pfc_ok2_OL SS2/updateSequencePhA/pol_vxn1/neg/SR ON/System Outputs1 ==

== system npc_controller/CONTROL/STATE-MACHINE/CPU_CONTROL_200_A2_precharge_pfc_ok2_OL SS2/updateSequencePhA/pol_vxn1/neg/SR ON/System Outputs2 ==

== system npc_controller/CONTROL/STATE-MACHINE/CPU_CONTROL_200_A2_precharge_pfc_ok2_OL SS2/updateSequencePhA/pol_vxn1/pos/SR Force to Low/System Outputs1 ==

== system npc_controller/CONTROL/STATE-MACHINE/CPU_CONTROL_200_A2_precharge_pfc_ok2_OL SS2/updateSequencePhA/pol_vxn1/pos/SR Force to Low/System Outputs2 ==

== system npc_controller/CONTROL/STATE-MACHINE/CPU_CONTROL_200_A2_precharge_pfc_ok2_OL SS2/updateSequencePhA/pol_vxn1/pos/SR ON/System Outputs1 ==

== system npc_controller/CONTROL/STATE-MACHINE/CPU_CONTROL_200_A2_precharge_pfc_ok2_OL SS2/updateSequencePhA/pol_vxn1/pos/SR ON/System Outputs2 ==

== system npc_controller/CONTROL/STATE-MACHINE/CPU_CONTROL_200_A2_precharge_pfc_ok2_OL SS2/updateSequencePhB/pol_vxn1/neg/SR OFF/System Outputs2 ==

== system npc_controller/CONTROL/STATE-MACHINE/CPU_CONTROL_200_A2_precharge_pfc_ok2_OL SS2/updateSequencePhB/pol_vxn1/neg/SR ON/System Outputs1 ==

== system npc_controller/CONTROL/STATE-MACHINE/CPU_CONTROL_200_A2_precharge_pfc_ok2_OL SS2/updateSequencePhB/pol_vxn1/pos/SR Force to Low/System Outputs2 ==

== system npc_controller/CONTROL/STATE-MACHINE/CPU_CONTROL_200_A2_precharge_pfc_ok2_OL SS2/updateSequencePhB/pol_vxn1/pos/SR ON/System Outputs1 ==

== system npc_controller/CONTROL/STATE-MACHINE/CPU_CONTROL_200_A2_precharge_pfc_ok2_OL SS2/updateSequencePhC/pol_vxn1/neg/SR OFF/System Outputs1 ==

== system npc_controller/CONTROL/STATE-MACHINE/CPU_CONTROL_200_A2_precharge_pfc_ok2_OL SS2/updateSequencePhC/pol_vxn1/neg/SR ON/System Outputs1 ==

== system npc_controller/CONTROL/STATE-MACHINE/CPU_CONTROL_200_A2_precharge_pfc_ok2_OL SS2/updateSequencePhC/pol_vxn1/pos/SR Force to Low/System Outputs2 ==

== system npc_controller/CONTROL/STATE-MACHINE/CPU_CONTROL_200_A2_precharge_pfc_ok2_OL SS2/updateSequencePhC/pol_vxn1/pos/SR ON/System Outputs1 ==

== system npc_controller/CONTROL/STATE-MACHINE/CPU_CONTROL_200_Vpk/configGrid/FORCE_TZ/1P/ALL_LEGS/System Outputs2 ==

== system npc_controller/CONTROL/STATE-MACHINE/CPU_CONTROL_200_Vpk/configGrid/FORCE_TZ/1P/LEG_A/System Outputs2 ==

== system npc_controller/CONTROL/STATE-MACHINE/CPU_CONTROL_200_Vpk/configGrid/FORCE_TZ/1P/LEG_B/System Outputs2 ==

== system npc_controller/CONTROL/STATE-MACHINE/CPU_CONTROL_200_Vpk/configGrid/FORCE_TZ/1P/LEG_C/System Outputs2 ==

== system npc_controller/CONTROL/STATE-MACHINE/CPU_CONTROL_200_Vpk/updatePll3p/PLL/SRF_PLL/Integrator/Accumulation ==
  In1 : Inport  OutDataTypeStr=single
  Action Port : ActionPort
  Out : Outport  OutDataTypeStr=single
  wires:
  In1/1 -> Out/1

== system npc_controller/CONTROL/STATE-MACHINE/CPU_CONTROL_200_Vpk/updatePll3p/PLL/SRF_PLL/Integrator/Reset Integrator ==
  Action Port : ActionPort
  Constant1 : Constant  Value=0  OutDataTypeStr=single
  Out : Outport
  wires:
  Constant1/1 -> Out/1

== system npc_controller/CONTROL/STATE-MACHINE/CPU_CONTROL_400/configGrid/FORCE_TZ/1P/ALL_LEGS/System Outputs2 ==

== system npc_controller/CONTROL/STATE-MACHINE/CPU_CONTROL_400/configGrid/FORCE_TZ/1P/LEG_A/System Outputs2 ==

== system npc_controller/CONTROL/STATE-MACHINE/CPU_CONTROL_400/configGrid/FORCE_TZ/1P/LEG_B/System Outputs2 ==

== system npc_controller/CONTROL/STATE-MACHINE/CPU_CONTROL_400/configGrid/FORCE_TZ/1P/LEG_C/System Outputs2 ==

== system npc_controller/CONTROL/STATE-MACHINE/CPU_CONTROL_400/updatePll3p/PLL/SRF_PLL/Integrator/Accumulation ==
  In1 : Inport  OutDataTypeStr=single
  Action Port : ActionPort
  Out : Outport  OutDataTypeStr=single
  wires:
  In1/1 -> Out/1

== system npc_controller/CONTROL/STATE-MACHINE/CPU_CONTROL_400/updatePll3p/PLL/SRF_PLL/Integrator/Reset Integrator ==
  Action Port : ActionPort
  Constant1 : Constant  Value=0  OutDataTypeStr=single
  Out : Outport
  wires:
  Constant1/1 -> Out/1

== system npc_controller/CONTROL/STATE-MACHINE/CPU_CONTROL_400_A2_precharge_pfc_ok2_OL SS/configGrid/FORCE_TZ/1P/ALL_LEGS/System Outputs2 ==

== system npc_controller/CONTROL/STATE-MACHINE/CPU_CONTROL_400_A2_precharge_pfc_ok2_OL SS/configGrid/FORCE_TZ/1P/LEG_A/System Outputs2 ==

== system npc_controller/CONTROL/STATE-MACHINE/CPU_CONTROL_400_A2_precharge_pfc_ok2_OL SS/configGrid/FORCE_TZ/1P/LEG_B/System Outputs2 ==

== system npc_controller/CONTROL/STATE-MACHINE/CPU_CONTROL_400_A2_precharge_pfc_ok2_OL SS/configGrid/FORCE_TZ/1P/LEG_C/System Outputs2 ==

== system npc_controller/CONTROL/STATE-MACHINE/CPU_CONTROL_400_A2_precharge_pfc_ok2_OL SS/updatePll3p/PLL/SRF_PLL/Integrator/Accumulation ==
  In1 : Inport  OutDataTypeStr=single
  Action Port : ActionPort
  Out : Outport  OutDataTypeStr=single
  wires:
  In1/1 -> Out/1

== system npc_controller/CONTROL/STATE-MACHINE/CPU_CONTROL_400_A2_precharge_pfc_ok2_OL SS/updatePll3p/PLL/SRF_PLL/Integrator/Reset Integrator ==
  Action Port : ActionPort
  Constant1 : Constant  Value=0  OutDataTypeStr=single
  Out : Outport
  wires:
  Constant1/1 -> Out/1

== system npc_controller/CONTROL/STATE-MACHINE/CPU_CONTROL_400_A2_precharge_pfc_ok2_OL SS2/configGrid/FORCE_TZ/1P/ALL_LEGS/System Outputs2 ==

== system npc_controller/CONTROL/STATE-MACHINE/CPU_CONTROL_400_A2_precharge_pfc_ok2_OL SS2/configGrid/FORCE_TZ/1P/LEG_A/System Outputs2 ==

== system npc_controller/CONTROL/STATE-MACHINE/CPU_CONTROL_400_A2_precharge_pfc_ok2_OL SS2/configGrid/FORCE_TZ/1P/LEG_B/System Outputs2 ==

== system npc_controller/CONTROL/STATE-MACHINE/CPU_CONTROL_400_A2_precharge_pfc_ok2_OL SS2/configGrid/FORCE_TZ/1P/LEG_C/System Outputs2 ==

== system npc_controller/CONTROL/STATE-MACHINE/CPU_CONTROL_400_A2_precharge_pfc_ok2_OL SS2/updatePll3p/PLL/SRF_PLL/Integrator/Accumulation ==
  In1 : Inport  OutDataTypeStr=single
  Action Port : ActionPort
  Out : Outport  OutDataTypeStr=single
  wires:
  In1/1 -> Out/1

== system npc_controller/CONTROL/STATE-MACHINE/CPU_CONTROL_400_A2_precharge_pfc_ok2_OL SS2/updatePll3p/PLL/SRF_PLL/Integrator/Reset Integrator ==
  Action Port : ActionPort
  Constant1 : Constant  Value=0  OutDataTypeStr=single
  Out : Outport
  wires:
  Constant1/1 -> Out/1

== system npc_controller/CONTROL/STATE-MACHINE/CPU_CONTROL_400_A2_precharge_pfc_ok2_OL SS2/updateSequencePhA/pol_vxn1/neg/SR OFF/System Outputs1 ==

== system npc_controller/CONTROL/STATE-MACHINE/CPU_CONTROL_400_A2_precharge_pfc_ok2_OL SS2/updateSequencePhA/pol_vxn1/neg/SR OFF/System Outputs2 ==

== system npc_controller/CONTROL/STATE-MACHINE/CPU_CONTROL_400_A2_precharge_pfc_ok2_OL SS2/updateSequencePhA/pol_vxn1/neg/SR ON/System Outputs1 ==

== system npc_controller/CONTROL/STATE-MACHINE/CPU_CONTROL_400_A2_precharge_pfc_ok2_OL SS2/updateSequencePhA/pol_vxn1/neg/SR ON/System Outputs2 ==

== system npc_controller/CONTROL/STATE-MACHINE/CPU_CONTROL_400_A2_precharge_pfc_ok2_OL SS2/updateSequencePhA/pol_vxn1/pos/SR Force to Low/System Outputs1 ==

== system npc_controller/CONTROL/STATE-MACHINE/CPU_CONTROL_400_A2_precharge_pfc_ok2_OL SS2/updateSequencePhA/pol_vxn1/pos/SR Force to Low/System Outputs2 ==

== system npc_controller/CONTROL/STATE-MACHINE/CPU_CONTROL_400_A2_precharge_pfc_ok2_OL SS2/updateSequencePhA/pol_vxn1/pos/SR ON/System Outputs1 ==

== system npc_controller/CONTROL/STATE-MACHINE/CPU_CONTROL_400_A2_precharge_pfc_ok2_OL SS2/updateSequencePhA/pol_vxn1/pos/SR ON/System Outputs2 ==

== system npc_controller/CONTROL/STATE-MACHINE/CPU_CONTROL_400_A2_precharge_pfc_ok2_OL SS2/updateSequencePhB/pol_vxn1/neg/SR OFF/System Outputs2 ==

== system npc_controller/CONTROL/STATE-MACHINE/CPU_CONTROL_400_A2_precharge_pfc_ok2_OL SS2/updateSequencePhB/pol_vxn1/neg/SR ON/System Outputs1 ==

== system npc_controller/CONTROL/STATE-MACHINE/CPU_CONTROL_400_A2_precharge_pfc_ok2_OL SS2/updateSequencePhB/pol_vxn1/pos/SR Force to Low/System Outputs2 ==

== system npc_controller/CONTROL/STATE-MACHINE/CPU_CONTROL_400_A2_precharge_pfc_ok2_OL SS2/updateSequencePhB/pol_vxn1/pos/SR ON/System Outputs1 ==

== system npc_controller/CONTROL/STATE-MACHINE/CPU_CONTROL_400_A2_precharge_pfc_ok2_OL SS2/updateSequencePhC/pol_vxn1/neg/SR OFF/System Outputs1 ==

== system npc_controller/CONTROL/STATE-MACHINE/CPU_CONTROL_400_A2_precharge_pfc_ok2_OL SS2/updateSequencePhC/pol_vxn1/neg/SR ON/System Outputs1 ==

== system npc_controller/CONTROL/STATE-MACHINE/CPU_CONTROL_400_A2_precharge_pfc_ok2_OL SS2/updateSequencePhC/pol_vxn1/pos/SR Force to Low/System Outputs2 ==

== system npc_controller/CONTROL/STATE-MACHINE/CPU_CONTROL_400_A2_precharge_pfc_ok2_OL SS2/updateSequencePhC/pol_vxn1/pos/SR ON/System Outputs1 ==

== system npc_controller/CONTROL/STATE-MACHINE/CPU_CONTROL_750_A2_precharge_pfc_ok1/configGrid/FORCE_TZ/1P/ALL_LEGS/System Outputs2 ==

== system npc_controller/CONTROL/STATE-MACHINE/CPU_CONTROL_750_A2_precharge_pfc_ok1/configGrid/FORCE_TZ/1P/LEG_A/System Outputs2 ==

== system npc_controller/CONTROL/STATE-MACHINE/CPU_CONTROL_750_A2_precharge_pfc_ok1/configGrid/FORCE_TZ/1P/LEG_B/System Outputs2 ==

== system npc_controller/CONTROL/STATE-MACHINE/CPU_CONTROL_750_A2_precharge_pfc_ok1/configGrid/FORCE_TZ/1P/LEG_C/System Outputs2 ==

== system npc_controller/CONTROL/STATE-MACHINE/CPU_CONTROL_750_A2_precharge_pfc_ok1/updatePll3p/PLL/SRF_PLL/Integrator/Accumulation ==
  In1 : Inport  OutDataTypeStr=single
  Action Port : ActionPort
  Out : Outport  OutDataTypeStr=single
  wires:
  In1/1 -> Out/1

== system npc_controller/CONTROL/STATE-MACHINE/CPU_CONTROL_750_A2_precharge_pfc_ok1/updatePll3p/PLL/SRF_PLL/Integrator/Reset Integrator ==
  Action Port : ActionPort
  Constant1 : Constant  Value=0  OutDataTypeStr=single
  Out : Outport
  wires:
  Constant1/1 -> Out/1

== system npc_controller/CONTROL/STATE-MACHINE/CPU_CONTROL_750_A2_precharge_pfc_ok2_OL SS1/configGrid/FORCE_TZ/1P/ALL_LEGS/System Outputs2 ==

== system npc_controller/CONTROL/STATE-MACHINE/CPU_CONTROL_750_A2_precharge_pfc_ok2_OL SS1/configGrid/FORCE_TZ/1P/LEG_A/System Outputs2 ==

== system npc_controller/CONTROL/STATE-MACHINE/CPU_CONTROL_750_A2_precharge_pfc_ok2_OL SS1/configGrid/FORCE_TZ/1P/LEG_B/System Outputs2 ==

== system npc_controller/CONTROL/STATE-MACHINE/CPU_CONTROL_750_A2_precharge_pfc_ok2_OL SS1/configGrid/FORCE_TZ/1P/LEG_C/System Outputs2 ==

== system npc_controller/CONTROL/STATE-MACHINE/CPU_CONTROL_750_A2_precharge_pfc_ok2_OL SS1/updatePll3p/PLL/SRF_PLL/Integrator/Accumulation ==
  In1 : Inport  OutDataTypeStr=single
  Action Port : ActionPort
  Out : Outport  OutDataTypeStr=single
  wires:
  In1/1 -> Out/1

== system npc_controller/CONTROL/STATE-MACHINE/CPU_CONTROL_750_A2_precharge_pfc_ok2_OL SS1/updatePll3p/PLL/SRF_PLL/Integrator/Reset Integrator ==
  Action Port : ActionPort
  Constant1 : Constant  Value=0  OutDataTypeStr=single
  Out : Outport
  wires:
  Constant1/1 -> Out/1
